simulink library "modbus_lib"  (Simulink 7.8)
settings: Solver=ode45  StartTime=0.0  StopTime=10.0  RelTol=1e-3
values from neighbouring files (symbols this model uses):
  relay_sets = xlsread('relay_settings_10272015.xlsx')    [relays_settings_init.m]
  Ts = 80e-6    (= 8e-05)    [global_parameters.m]    (also in scopeBuffer.m)
undefined symbols (not defined in the file or in its folder): angle_threshold, dF_threshold, DiscIntNeverNeededParam, dV_threshold, IOC, TOC, V, VRMSLL
libraries: simulink x24, powerlib_extras x20, powerlib x14, modbus_lib x6, simulink_extras x5, lib_Timer_Counter x4, rtio_generic_modbus x3, dspsigops x2
(part 1 of 2)
settings Model: Creator=RE25624  LastModifiedBy=re25624

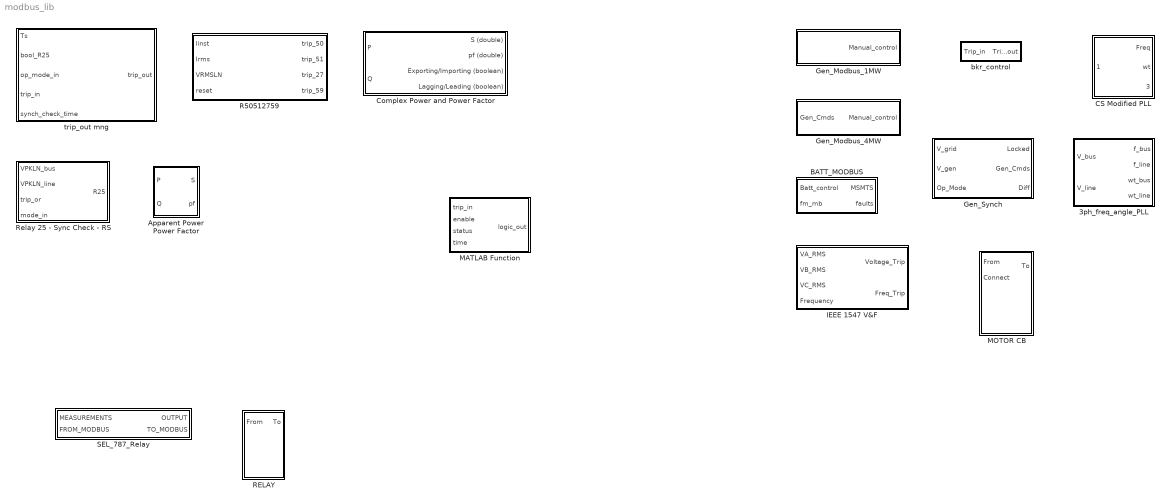
== system modbus_lib ==
  3ph_freq_angle_PLL : Subsystem
  Apparent Power Power Factor : Subsystem
  BATT_MODBUS : Subsystem
  CS Modified PLL : Subsystem  DialogController=POWERSYS.PowerSysDialog  mask(Discrete 3-phase PLL){Fmin=50, Par_Init=[0 60], ParK=[ 180 3200 1 ], Ts=Ts, AGC=off}
      mask prompts: Fmin "Minimum frequency (Hz):"; Par_Init "Initial inputs:[ Phase(degrees)   Frequency(Hz) ]"; ParK "Regulator gains [ Kp  Ki  Kd ]"; Ts "Sample time:"; AGC "Enable Automatic Gain Control"
      mask help:
      | This Phase Locked Loop (PLL) system can be used  to synchronize on a set of variable frequency, three-phase sinusoidal signals. If the Automatic Gain Control is enabled, the input (phase error) of the PLL regulator is scaled according to the input signals magnitude.
      |
      | For optimal performance, the following settings are recommended:
      |   [ Kp Ki  Kd ] = [ 180  3200  1 ]
      |   "Enable Automatic Gain Control" checked
      |
      | Input 1: Vector containing the normalized three-phase signals [Va Vb Vc]
      | Output 1:  Measured frequency (Hz) = w/(2pi)
      | Output 2:  Ramp w.t varying between  0 and 2*pi,
      |      synchronized on zero crossings of the fundamental (positive-sequence) of phase A.
      | Output 3: Vector [sin(wt) cos(wt)]
      mask init:
      | Kp=ParK(1);
      | Ki=ParK(2);
      | if length(ParK)==2
      |     Kd=0;
      | else
      |     Kd=ParK(3);
      | end    
      | Phase_Init=Par_Init(1);
      | Finit=Par_Init(2);
      | power_initmask();
      settings: OpenFcn=power_openblockproxy();
      mask Display: disp('')
  Complex Power and Power Factor : Subsystem
  Gen_Modbus_1MW : Subsystem
  Gen_Modbus_4MW : Subsystem
  Gen_Synch : Subsystem
  IEEE 1547 V&F : Subsystem  mask{V=VRMSLL, OF1=2, OF2=0.16, OV1=13, OV2=0.16, UF1=0.16, UF2=2, UV1=0.16, UV2=11, UV3=21}
      mask prompts: V "VoltageLL_RMS"; OF1 "OF1 (>60.5 Hz)"; OF2 "OF2 (>62 Hz)"; OV1 "OV1 (110% <V< 120% Vnom"; OV2 "OV2 (120% Vnom)"; UF1 "UF1 (<57 Hz)"; UF2 "UF2 (<59.5 Hz)"; UV1 "UV1 (<45% Vnom)"; UV2 "UV2 (45%<V<60% Vnom)"; UV3 "UV3 (60%<V<88% Vnom)"
      mask help:
      | This block implements interconnection system response according to IEEE Std. 1547-2014a.
      |
      | Fields to be filled are clearing times in seconds.
  MATLAB Function : MATLAB Function  TreatAsAtomicUnit=on
  MOTOR CB : Subsystem  mask(Breaker){Ts=Ts}
      mask prompts: Ts "Sampling Time [Sec]"
      mask help:
      | This block simulates the open/close behavior of a breaker. The logic (1-closed; 0-open) of operation is provided via external relay-blocks.
      | The breaker model also facilitates the system measurements for all logic functions to operate.
      | The connectivity convention adopted for this block is as follows: ABC indicates the “entry-point” or line, and the abc indicates the “exit-point” or bus.
  R50512759 : Subsystem  mask(Relays 50-51-27-59){VRMSLL=VRMSLL, IOC=IOC, TOC=TOC, Ts=Ts}
      mask prompts: VRMSLL "Nominal Voltage [VRMSLL]"; IOC "IOC Setting [A]"; TOC "TOC Setting [A]"; Ts "Sampling Time [Sec]"
      mask help:
      | This block simulates the behavior of the following relay functions:
      | 1) Instantaneous overcurrent (50)
      | 2) AC inverse time overcurrent (51)
      | 3) Undervoltage (27)
      | 4) Overvoltage (59)
      | It is not suitable for instantaneous earth current relaying.
      | The model neglects the influence CTs since only the logics of the relay are required or the current effort.
  RELAY : Subsystem  mask(Breaker){Ts=Ts}
      mask prompts: Ts "Sampling Time [Sec]"
      mask help:
      | This block simulates the open/close behavior of a breaker. The logic (1-closed; 0-open) of operation is provided via external relay-blocks.
      | The breaker model also facilitates the system measurements for all logic functions to operate.
      | The connectivity convention adopted for this block is as follows: ABC indicates the “entry-point” or line, and the abc indicates the “exit-point” or bus.
  Relay 25 - Sync Check - RS : Subsystem  mask{VRMSLL=VRMSLL, Ts=Ts, dV_threshold=dV_threshold, angle_threshold=angle_threshold, dF_threshold=dF_threshold}
      mask prompts: VRMSLL "Nominal Voltage [VRMSLL]"; Ts "Sampling Time [Sec]"; dV_threshold "Percent Voltage Threshold [%]"; angle_threshold "Angle Threshold [degress]"; dF_threshold "Frequency Threshold [Hz]"
  SEL_787_Relay : Subsystem  mask(Relay Model){bkrCtrl_enable=0, bkrCtrl_status=1, settings=[relay_sets(1, :)], Ts=Ts}
      mask prompts: bkrCtrl_enable "Enable - manual breaker control"; bkrCtrl_status "Status - manual breaker control"; settings "Relay Settings [Vnom(VRMSLL) IOC(A) TOC(A) dV(%)  dA(degrees)  dF(Hz)]"; Ts "Sampling Time [Sec]"
      mask help:
      | * The simulated relay functions are the following: synchronizing or synchronism-check (25), phase instantaneous overcurrent (50P), AC inverse time overcurrent (51P), undervoltage relay (27), and overvoltage relay (59).
      | * Modbus communication arranged to approximate SEL-787
      | * Locked-out only enabled for functions (50), (51)
      | * Over/undervoltage settings are set to +-15% of nominal voltage
      | * Manual breaker status: [1-closed, 0-open]
      mask init:
      | VRMSLL = settings(1);
      | IOC = settings(2);
      | TOC = settings(3);
      | dV_threshold = settings(4)/100;
      | angle_threshold = settings(5);
      | dF_threshold = settings(6);
  bkr_control : Subsystem  mask(Breaker control){enable=0, status=1}
      mask prompts: status "Breaker status: [1-closed, 0-open]"
      mask help: Allows the user to select which trip signal will be received at the breaker.
  trip_out mng : MATLAB Function  TreatAsAtomicUnit=on

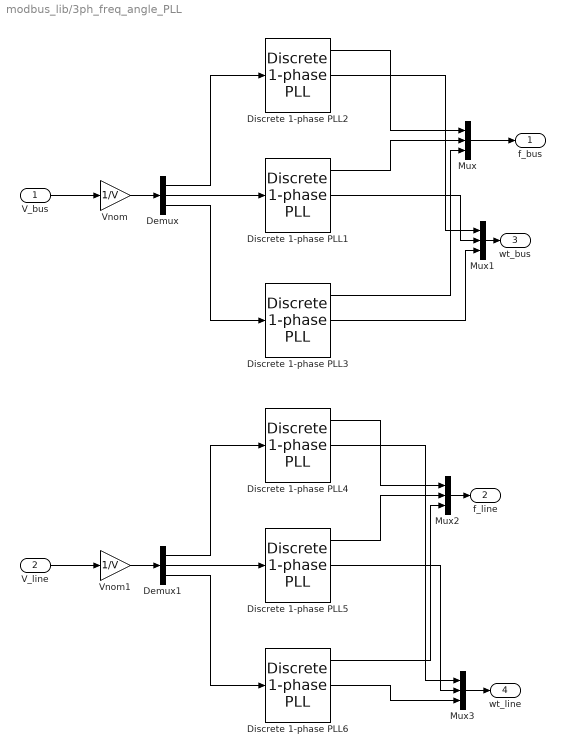
== system modbus_lib/3ph_freq_angle_PLL ==
  V_bus : Inport
  V_line : Inport  Port=2
  Demux : Demux  Outputs=3
  Demux1 : Demux  Outputs=3
  Discrete 1-phase PLL{1..6} (6 alike) : powerlib_extras/Discrete  Control Blocks/Discrete 1-phase PLL  Fmin=45  Par_Init=[0 60]  ParK=[ 180 3200 1]  Ts=50e-6  AGC=on
  Mux{,1..3} (4 alike) : Mux  Inputs=3
  Vnom : Gain  Gain=1/V
  Vnom1 : Gain  Gain=1/V
  f_bus : Outport
  f_line : Outport  Port=2
  wt_bus : Outport  Port=3
  wt_line : Outport  Port=4
  wires:
  V_bus/1 -> Vnom/1
  Mux3/1 -> wt_line/1
  Mux2/1 -> f_line/1
  Discrete 1-phase PLL6/2 -> Mux3/3
  Discrete 1-phase PLL5/2 -> Mux3/2
  Discrete 1-phase PLL4/2 -> Mux3/1
  Discrete 1-phase PLL5/1 -> Mux2/2
  Discrete 1-phase PLL6/1 -> Mux2/3
  Discrete 1-phase PLL4/1 -> Mux2/1
  Mux1/1 -> wt_bus/1
  Discrete 1-phase PLL3/2 -> Mux1/3
  Discrete 1-phase PLL1/2 -> Mux1/2
  Discrete 1-phase PLL2/2 -> Mux1/1
  Mux/1 -> f_bus/1
  Discrete 1-phase PLL3/1 -> Mux/3
  Discrete 1-phase PLL1/1 -> Mux/2
  Discrete 1-phase PLL2/1 -> Mux/1
  Demux/3 -> Discrete 1-phase PLL3/1
  Demux/2 -> Discrete 1-phase PLL1/1
  Demux/1 -> Discrete 1-phase PLL2/1
  Demux1/3 -> Discrete 1-phase PLL6/1
  Demux1/2 -> Discrete 1-phase PLL5/1
  Demux1/1 -> Discrete 1-phase PLL4/1
  Vnom1/1 -> Demux1/1
  Vnom/1 -> Demux/1
  V_line/1 -> Vnom1/1

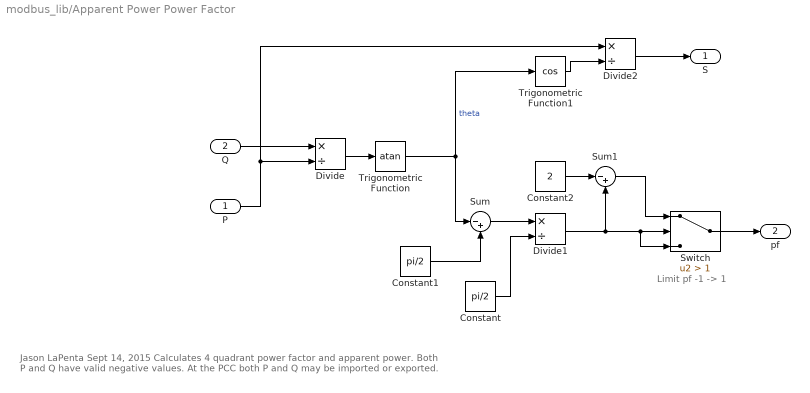
== system modbus_lib/Apparent Power Power Factor ==
  note: Limit pf -1 -> 1
  note: Jason LaPenta
      | Sept 14, 2015
      |
      | Calculates 4 quadrant power factor and apparent power.
      | Both P and Q have valid negative values. At the PCC
      | both P and Q may be imported or exported.
  P : Inport
  Q : Inport  Port=2
  Constant : Constant  Value=pi/2
  Constant1 : Constant  Value=pi/2
  Constant2 : Constant  Value=2
  Divide : Product  Inputs=*/
  Divide1 : Product  Inputs=*/
  Divide2 : Product  Inputs=*/
  Sum : Sum  Inputs=|-+
  Sum1 : Sum  Inputs=|-+
  Switch : Switch  Criteria=u2 > Threshold  Threshold=1
  Trigonometric Function : Trigonometry  Operator=atan
  Trigonometric Function1 : Trigonometry  Operator=cos
  S : Outport
  pf : Outport  Port=2
  wires:
  Switch/1 -> pf/1
  Constant2/1 -> Sum1/1
  Sum1/1 -> Switch/1
  Divide1/1 -> Switch/3, Switch/2, Sum1/2
  Sum/1 -> Divide1/1
  Constant1/1 -> Sum/2
  Divide2/1 -> S/1
  Trigonometric Function1/1 -> Divide2/2
  Constant/1 -> Divide1/2
  Trigonometric Function/1 -> Sum/1, Trigonometric Function1/1  "theta"
  Divide/1 -> Trigonometric Function/1
  P/1 -> Divide2/1, Divide/2
  Q/1 -> Divide/1

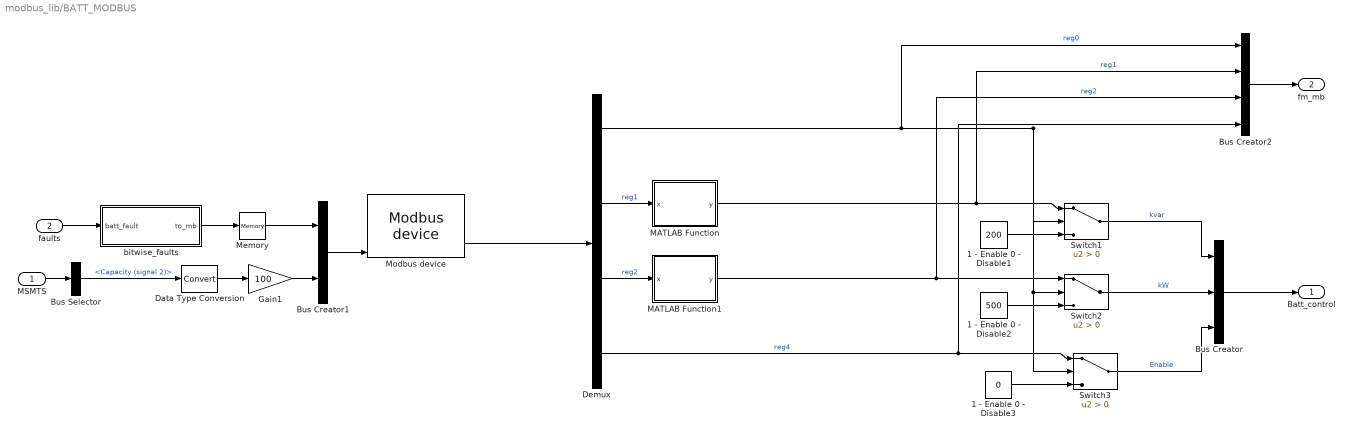
== system modbus_lib/BATT_MODBUS ==
  MSMTS : Inport
  faults : Inport  Port=2
  1 - Enable 0 - Disable1 : Constant  Value=200
  1 - Enable 0 - Disable2 : Constant  Value=500
  1 - Enable 0 - Disable3 : Constant  Value=0
  Bus Creator : BusCreator  Inputs=3
  Bus Creator1 : BusCreator  Inputs=2
  Bus Creator2 : BusCreator
  Bus Selector : BusSelector  OutputSignals=Capacity (signal 2)
  Data Type Conversion : DataTypeConversion
  Demux : Demux
  Gain1 : Gain  Gain=100
  MATLAB Function : MATLAB Function  TreatAsAtomicUnit=on
  MATLAB Function1 : MATLAB Function  TreatAsAtomicUnit=on
  Memory : Memory
  Modbus device : rtio_generic_modbus/Modbus device  conf_name=batt_slave_cfg.opal  conf_name_mask=batt_slave_cfg.xls  sample_time=Ts
  Switch1 : Switch  Criteria=u2 > Threshold
  Switch2 : Switch  Criteria=u2 > Threshold
  Switch3 : Switch  Criteria=u2 > Threshold
  bitwise_faults : Subsystem
  Batt_control : Outport
  fm_mb : Outport  Port=2
  wires:
  MATLAB Function/1(y) -> Bus Creator2/2, Switch1/1  "reg1"
  MATLAB Function1/1(y) -> Bus Creator2/3, Switch2/1  "reg2"
  Memory/1 -> Bus Creator1/1
  faults/1 -> bitwise_faults/1(batt_fault)
  bitwise_faults/1(to_mb) -> Memory/1
  Bus Creator2/1 -> fm_mb/1
  Gain1/1 -> Bus Creator1/2
  Bus Creator1/1 -> Modbus device/4
  Data Type Conversion/1 -> Gain1/1
  Bus Selector/1 -> Data Type Conversion/1  "<Capacity (signal 2)>"
  MSMTS/1 -> Bus Selector/1
  Bus Creator/1 -> Batt_control/1
  Switch3/1 -> Bus Creator/3  "Enable"
  Switch2/1 -> Bus Creator/2  "kW"
  Switch1/1 -> Bus Creator/1  "kvar"
  Demux/1 -> Bus Creator2/1, Switch3/2, Switch2/2, Switch1/2  "reg0"
  Demux/4 -> Bus Creator2/4, Switch3/1  "reg4"
  Demux/3 -> MATLAB Function1/1(x)  "reg2"
  Demux/2 -> MATLAB Function/1(x)  "reg1"
  1 - Enable 0 - Disable3/1 -> Switch3/3
  1 - Enable 0 - Disable2/1 -> Switch2/3
  1 - Enable 0 - Disable1/1 -> Switch1/3
  Modbus device/2 -> Demux/1

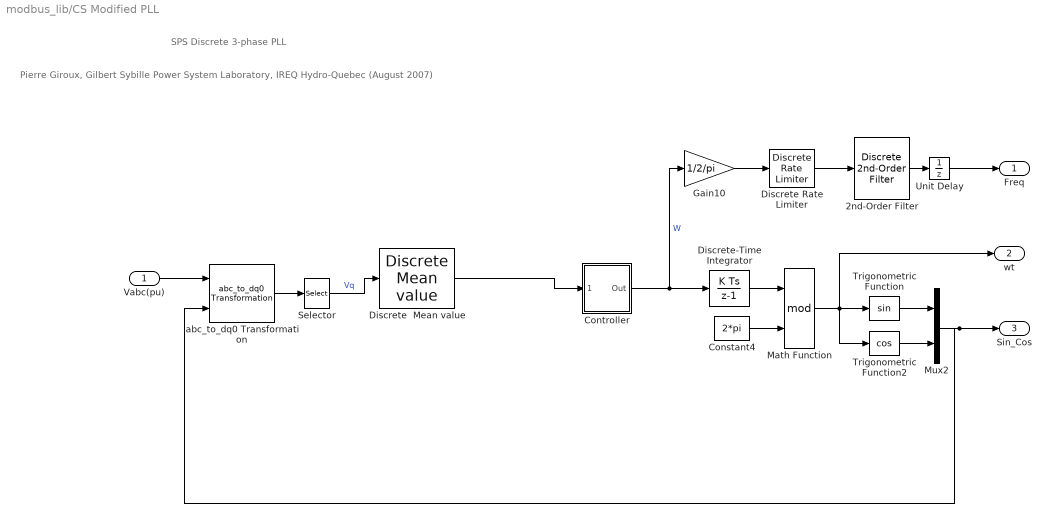
== system modbus_lib/CS Modified PLL ==
  note: Pierre Giroux, Gilbert Sybille
      | Power System Laboratory, IREQ
      | Hydro-Quebec
      | (August 2007)
  note: SPS Discrete 3-phase PLL
  Vabc(pu) : Inport  PortDimensions=3
  2nd-Order Filter : powerlib_extras/Discrete  Control Blocks/Discrete  2nd-Order Filter  FilterType=Lowpass  Fo=25  Zeta=0.707  Ts=Ts  Initialize=on  Vac_Init=[0 0 Finit]  Vdc_Init=Finit  PlotResponse=off  param1=[1 500 0.1]
  Constant4 : Constant  Value=2*pi
  Controller : Subsystem  mask(Discrete PID Controller){Kp=Kp, Ki=Ki, Kd=Kd, Par_Limits=[10000 0], Init=2*pi*Finit, Ts=Ts}
      mask prompts: Kp "Proportional gain (Kp):"; Ki "Integral gain (Ki):"; Kd "Derivative gain (Kd):"; Par_Limits "Output limits: [ Upper   Lower ]"; Init "Output initial value:"; Ts "Sample time:"
      mask help: This block implements a discrete PID controller.
      mask init:
      | UpperLimit=Par_Limits(1);
      | LowerLimit=Par_Limits(2);
      | power_initmask();
      settings: OpenFcn=power_openblockproxy();
      mask Display: disp('PID');
  Discrete Rate Limiter : powerlib_extras/Discrete  Control Blocks/Discrete Rate Limiter  R=12  F=-12  Vinit=Finit  Ts=Ts
  Discrete  Mean value : powerlib_extras/Discrete Measurements/Discrete  Mean value  Freq=60  Vinit=0  Ts=Ts
  Discrete-Time Integrator : DiscreteIntegrator  InitialCondition=Phase_Init*pi/180  SampleTime=Ts  ICPrevOutput=DiscIntNeverNeededParam  ICPrevScaledInput=DiscIntNeverNeededParam
  Gain10 : Gain  Gain=1/2/pi  SaturateOnIntegerOverflow=on  OutDataTypeStr=Inherit: Same as input  ParamDataTypeStr=Inherit: Same as input
  Math Function : Math  Operator=mod  SaturateOnIntegerOverflow=on
  Mux2 : Mux  Inputs=2
  Selector : Selector  InputPortWidth=3  IndexOptions=Index vector (dialog)  Indices=2  OutputSizes=1
  Trigonometric Function : Trigonometry
  Trigonometric Function2 : Trigonometry  Operator=cos
  Unit Delay : UnitDelay  X0=Finit  SampleTime=Ts
  abc_to_dq0 Transformation : powerlib_extras/Measurements/abc_to_dq0 Transformation
  Freq : Outport
  wt : Outport  Port=2
  Sin_Cos : Outport  Port=3
  wires:
  Selector/1 -> Discrete  Mean value/1  "Vq"
  2nd-Order Filter/1 -> Unit Delay/1
  Unit Delay/1 -> Freq/1
  Discrete Rate Limiter/1 -> 2nd-Order Filter/1
  Gain10/1 -> Discrete Rate Limiter/1
  Mux2/1 -> Sin_Cos/1, abc_to_dq0 Transformation/2
  Trigonometric Function2/1 -> Mux2/2
  Trigonometric Function/1 -> Mux2/1
  Math Function/1 -> Trigonometric Function/1, wt/1, Trigonometric Function2/1
  Discrete-Time Integrator/1 -> Math Function/1
  Constant4/1 -> Math Function/2
  abc_to_dq0 Transformation/1 -> Selector/1
  Vabc(pu)/1 -> abc_to_dq0 Transformation/1
  Controller/1(Out) -> Discrete-Time Integrator/1, Gain10/1  "W"
  Discrete  Mean value/1 -> Controller/1(Error)

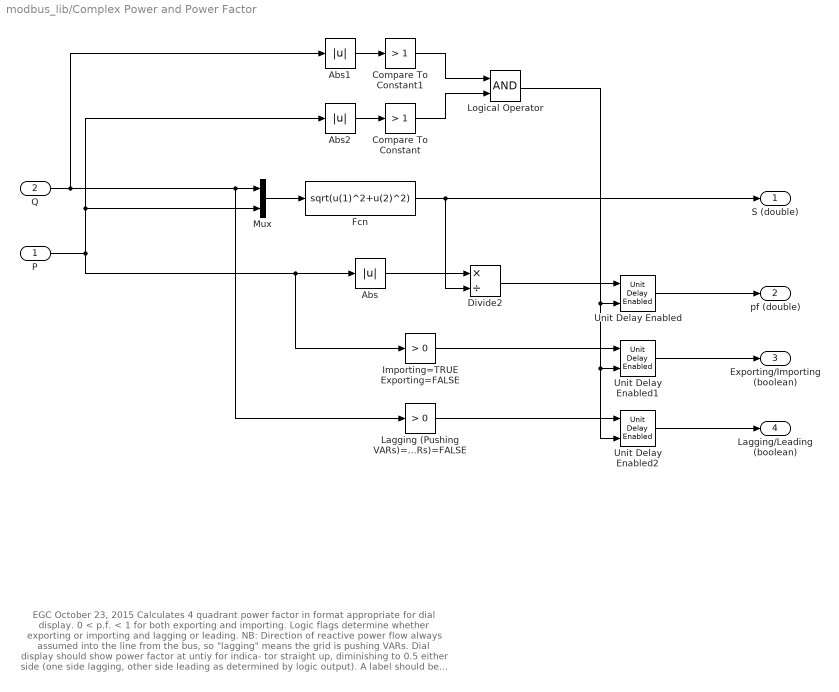
== system modbus_lib/Complex Power and Power Factor ==
  note: EGC
      | October 23, 2015
      |
      | Calculates 4 quadrant power factor in format appropriate
      | for dial display.  0 < p.f. < 1 for both exporting and
      | importing.  Logic flags determine whether exporting or
      | importing and lagging or leading.  NB:  Direction of
      | reactive power flow always assumed into the line from the
      | bus, so "lagging" means the grid is pushing VARs.
      |
      | Dial display should show power factor at untiy for indica-
      | tor straight up, diminishing to 0.5 either side (one side
      | lagging, other side leading as determined by logic output).
      | A label should be used to display EXPORTING or IMPORTING
      | based on logic output.
  P : Inport
  Q : Inport  Port=2
  Abs : Abs
  Abs1 : Abs
  Abs2 : Abs
  Compare To Constant : simulink/Logic and Bit Operations/Compare To Constant  relop=>  const=1  OutDataTypeStr=uint8
  Compare To Constant1 : simulink/Logic and Bit Operations/Compare To Constant  relop=>  const=1  OutDataTypeStr=uint8
  Divide2 : Product  Inputs=*/
  Fcn : Fcn  Expr=sqrt(u(1)^2+u(2)^2)
  Importing=TRUE Exporting=FALSE : simulink/Logic and Bit Operations/Compare To Constant  relop=>  const=0  OutDataTypeStr=boolean
  Lagging (Pushing VARs)=TRUE Leading (Pulling VARs)=FALSE : simulink/Logic and Bit Operations/Compare To Constant  relop=>  const=0  OutDataTypeStr=boolean
  Logical Operator : Logic  AllPortsSameDT=off  OutDataTypeStr=boolean
  Mux : Mux  Inputs=2
  Unit Delay Enabled : simulink/Additional Math & Discrete/Additional Discrete/Unit Delay Enabled  vinit=1  tsamp=-1
  Unit Delay Enabled1 : simulink/Additional Math & Discrete/Additional Discrete/Unit Delay Enabled  vinit=1  tsamp=-1
  Unit Delay Enabled2 : simulink/Additional Math & Discrete/Additional Discrete/Unit Delay Enabled  vinit=1  tsamp=-1
  S (double) : Outport
  pf (double) : Outport  Port=2
  Exporting/Importing (boolean) : Outport  Port=3
  Lagging/Leading (boolean) : Outport  Port=4
  wires:
  Fcn/1 -> Divide2/2, S (double)/1
  P/1 -> Abs/1, Importing=TRUE Exporting=FALSE/1, Mux/2, Abs2/1
  Q/1 -> Mux/1, Lagging (Pushing VARs)=TRUE Leading (Pulling VARs)=FALSE/1, Abs1/1
  Mux/1 -> Fcn/1
  Abs/1 -> Divide2/1
  Divide2/1 -> Unit Delay Enabled/1
  Unit Delay Enabled/1 -> pf (double)/1
  Importing=TRUE Exporting=FALSE/1 -> Unit Delay Enabled1/1
  Unit Delay Enabled1/1 -> Exporting/Importing (boolean)/1
  Lagging (Pushing VARs)=TRUE Leading (Pulling VARs)=FALSE/1 -> Unit Delay Enabled2/1
  Unit Delay Enabled2/1 -> Lagging/Leading (boolean)/1
  Abs2/1 -> Compare To Constant/1
  Abs1/1 -> Compare To Constant1/1
  Compare To Constant1/1 -> Logical Operator/1
  Compare To Constant/1 -> Logical Operator/2
  Logical Operator/1 -> Unit Delay Enabled/2, Unit Delay Enabled1/2, Unit Delay Enabled2/2

== system modbus_lib/Gen_Modbus_1MW ==
  note: This function is an attempt to substitute the switches
  Bus Creator : BusCreator  Inputs=6
  Demux : Demux  Outputs=7
  Gain : Gain  Gain=1/100
  MATLAB Function : MATLAB Function  TreatAsAtomicUnit=on
  Modbus device : rtio_generic_modbus/Modbus device  conf_name=none  conf_name_mask=gen_slave_cfg2.xls  sample_time=Ts
  Manual_control : Outport
  wires:
  Gain/1 -> Demux/1
  Modbus device/2 -> Gain/1
  Demux/1 -> MATLAB Function/1(Select_mb)
  Demux/2 -> MATLAB Function/2(P_mb)
  Demux/3 -> MATLAB Function/3(Q_mb)
  Demux/4 -> MATLAB Function/4(V_mb)
  Demux/5 -> MATLAB Function/5(F_mb)
  Demux/6 -> MATLAB Function/6(Mode_mb)
  Demux/7 -> MATLAB Function/7(Enable_mb)
  Bus Creator/1 -> Manual_control/1
  MATLAB Function/1(P) -> Bus Creator/1  "P"
  MATLAB Function/2(Q) -> Bus Creator/2  "Q"
  MATLAB Function/3(V) -> Bus Creator/3  "V"
  MATLAB Function/4(F) -> Bus Creator/4  "F"
  MATLAB Function/5(Mode) -> Bus Creator/5  "Mode"
  MATLAB Function/6(Enable) -> Bus Creator/6  "Enable"

== system modbus_lib/Gen_Modbus_4MW ==
  note: This function is an attempt to substitute the switches
  Gen_Cmds : Inport
  Bus Creator : BusCreator  Inputs=6
  Demux : Demux  Outputs=7
  Gain : Gain  Gain=1/100
  MATLAB Function : MATLAB Function  TreatAsAtomicUnit=on
  Modbus device : rtio_generic_modbus/Modbus device  conf_name=gen_slave_cfg.opal  conf_name_mask=gen_slave_cfg.xls  sample_time=Ts
  Manual_control : Outport
  wires:
  Gain/1 -> Demux/1
  Demux/1 -> MATLAB Function/1(Select_mb)
  Demux/2 -> MATLAB Function/2(P_mb)
  Demux/3 -> MATLAB Function/3(Q_mb)
  Demux/4 -> MATLAB Function/4(V_mb)
  Demux/5 -> MATLAB Function/5(F_mb)
  Demux/6 -> MATLAB Function/6(Mode_mb)
  Demux/7 -> MATLAB Function/7(Enable_mb)
  Bus Creator/1 -> Manual_control/1
  MATLAB Function/1(P) -> Bus Creator/1  "P"
  MATLAB Function/2(Q) -> Bus Creator/2  "Q"
  MATLAB Function/3(V) -> Bus Creator/3  "V"
  MATLAB Function/4(F) -> Bus Creator/4  "F"
  MATLAB Function/5(Mode) -> Bus Creator/5  "Mode"
  MATLAB Function/6(Enable) -> Bus Creator/6  "Enable"
  Modbus device/2 -> Gain/1
  Gen_Cmds/1 -> MATLAB Function/8(gen_cmds)

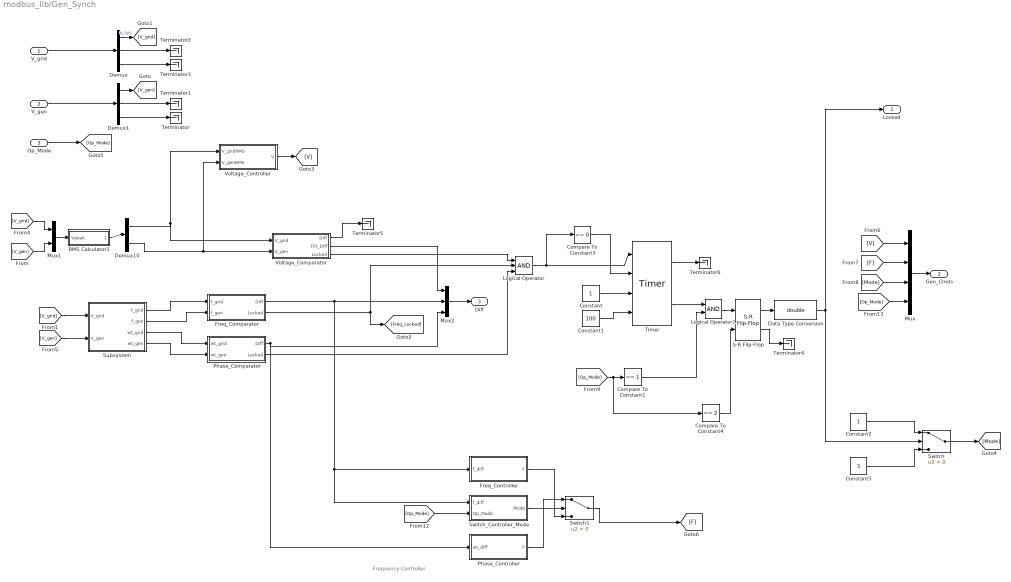
== system modbus_lib/Gen_Synch ==
  note: Frequency Controller
  V_grid : Inport
  V_gen : Inport  Port=2
  Op_Mode : Inport  Port=3
  Compare To Constant1 : simulink/Logic and Bit Operations/Compare To Constant  relop===  const=1  OutDataTypeStr=boolean
  Compare To Constant3 : simulink/Logic and Bit Operations/Compare To Constant  relop===  const=0  OutDataTypeStr=uint8
  Compare To Constant4 : simulink/Logic and Bit Operations/Compare To Constant  relop===  const=2  OutDataTypeStr=boolean
  Constant : Constant
  Constant1 : Constant  Value=100
  Constant2 : Constant
  Constant3 : Constant  Value=3
  Data Type Conversion : DataTypeConversion  OutDataTypeStr=double
  Demux : Demux  Outputs=3
  Demux1 : Demux  Outputs=3
  Demux10 : Demux  Outputs=2
  Freq_Comparator : Subsystem
  Freq_Controller : Subsystem
  Logical Operator : Logic  Inputs=3  AllPortsSameDT=off  OutDataTypeStr=boolean
  Logical Operator1 : Logic  AllPortsSameDT=off  OutDataTypeStr=boolean
  Mux : Mux
  Mux1 : Mux  Inputs=2
  Mux2 : Mux  Inputs=3
  Phase_Comparator : Subsystem
  Phase_Controller : Subsystem
  RMS Calculator3 : Subsystem
  S-R Flip-Flop : simulink_extras/Flip Flops/S-R Flip-Flop  initial_condition=0
  Subsystem : Subsystem
  Switch : Switch  Criteria=u2 > Threshold
  Switch1 : Switch  Criteria=u2 > Threshold
  Switch_Controller_Mode : Subsystem
  Terminator{,1..6} (7 alike) : Terminator
  Timer : lib_Timer_Counter/Timer
  Voltage_Comparator : Subsystem
  Voltage_Controller : Subsystem
  Locked : Outport
  Gen_Cmds : Outport  Port=2  PortDimensions=4
  Diff : Outport  Port=3
  wires:
  Phase_Comparator/1(Diff) -> Mux2/3, Phase_Controller/1(wt_diff)
  Freq_Comparator/1(Diff) -> Mux2/2, Freq_Controller/1(f_diff), Switch_Controller_Mode/1(f_diff)
  Voltage_Comparator/2(Filt_Diff) -> Mux2/1
  [V_gen] -> Subsystem/2(V_gen)
  [V_grid] -> Subsystem/1(V_grid)
  Demux/1 -> [V_grid]  "a_sys"
  Demux1/1 -> [V_gen]
  Data Type Conversion/1 -> Switch/2, Locked/1
  S-R Flip-Flop/1 -> Data Type Conversion/1
  Logical Operator/1 -> Compare To Constant3/1, Timer/1
  Compare To Constant3/1 -> Timer/2
  Constant1/1 -> Timer/4
  Constant/1 -> Timer/3
  Phase_Comparator/2(Locked) -> Logical Operator/3
  Freq_Comparator/2(Locked) -> Logical Operator/2, [Freq_Locked]
  Voltage_Comparator/3(Locked) -> Logical Operator/1
  Subsystem/4(wt_gen) -> Phase_Comparator/2(wt_gen)
  Subsystem/3(wt_grid) -> Phase_Comparator/1(wt_grid)
  Subsystem/2(f_gen) -> Freq_Comparator/2(f_gen)
  Subsystem/1(f_grid) -> Freq_Comparator/1(f_grid)
  V_gen/1 -> Demux1/1
  V_grid/1 -> Demux/1
  Constant2/1 -> Switch/1
  Constant3/1 -> Switch/3
  Switch/1 -> [Mode]
  Mux/1 -> Gen_Cmds/1
  [V] -> Mux/1
  [Mode] -> Mux/3
  [F] -> Mux/2
  Timer/2 -> Logical Operator1/1
  Compare To Constant1/1 -> Logical Operator1/2
  Mux2/1 -> Diff/1
  Switch1/1 -> [F]
  Switch_Controller_Mode/1(Mode) -> Switch1/2
  Op_Mode/1 -> [Op_Mode]
  [Op_Mode] -> Compare To Constant1/1, Compare To Constant4/1
  Logical Operator1/1 -> S-R Flip-Flop/1
  Compare To Constant4/1 -> S-R Flip-Flop/2
  [Op_Mode] -> Mux/4
  Voltage_Controller/1(V) -> [V]
  Freq_Controller/1(F) -> Switch1/3
  Phase_Controller/1(F) -> Switch1/1
  [Op_Mode] -> Switch_Controller_Mode/2(Op_Mode)
  Demux1/2 -> Terminator1/1
  Demux1/3 -> Terminator/1
  Demux/2 -> Terminator2/1
  Demux/3 -> Terminator3/1
  S-R Flip-Flop/2 -> Terminator4/1
  Voltage_Comparator/1(Diff) -> Terminator5/1
  Demux10/2 -> Voltage_Comparator/2(V_gen), Voltage_Controller/2(V_genRMS)
  Mux1/1 -> RMS Calculator3/1(Vpeak)
  RMS Calculator3/1(VRMSLL) -> Demux10/1
  [V_grid] -> Mux1/1
  [V_gen] -> Mux1/2
  Demux10/1 -> Voltage_Controller/1(V_gridRMS), Voltage_Comparator/1(V_grid)
  Timer/1 -> Terminator6/1

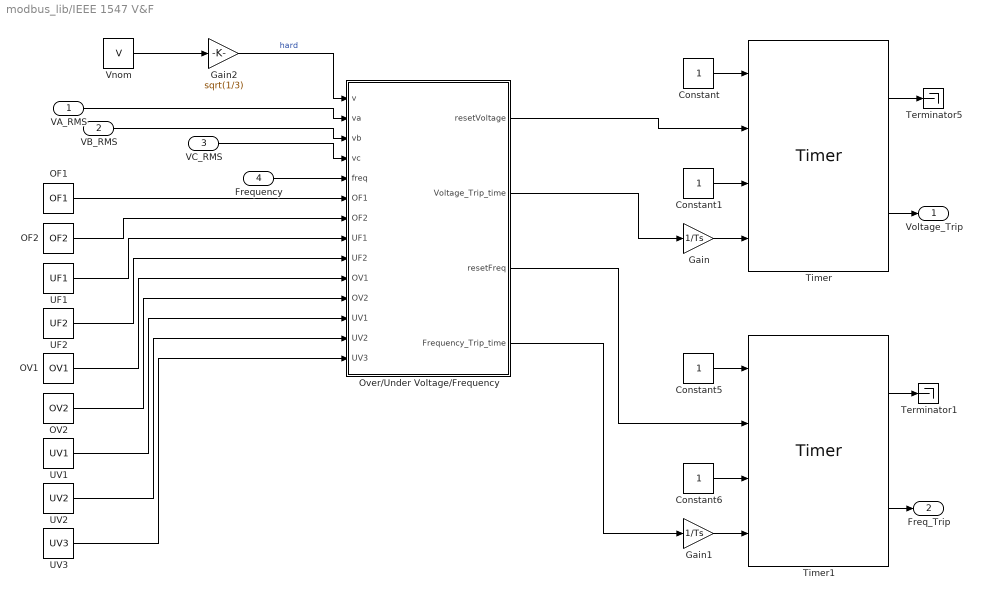
== system modbus_lib/IEEE 1547 V&F ==
  VA_RMS : Inport
  VB_RMS : Inport  Port=2
  VC_RMS : Inport  Port=3
  Frequency : Inport  Port=4
  Constant{,1,5..6} (4 alike) : Constant
  Gain : Gain  Gain=1/Ts
  Gain1 : Gain  Gain=1/Ts
  Gain2 : Gain  Gain=sqrt(1/3)
  OF1 : Constant  Value=OF1
  OF2 : Constant  Value=OF2
  OV1 : Constant  Value=OV1
  OV2 : Constant  Value=OV2
  Over/Under Voltage/Frequency : MATLAB Function  TreatAsAtomicUnit=on
  Terminator1 : Terminator
  Terminator5 : Terminator
  Timer : lib_Timer_Counter/Timer
  Timer1 : lib_Timer_Counter/Timer
  UF1 : Constant  Value=UF1
  UF2 : Constant  Value=UF2
  UV1 : Constant  Value=UV1
  UV2 : Constant  Value=UV2
  UV3 : Constant  Value=UV3
  Vnom : Constant  Value=V
  Voltage_Trip : Outport
  Freq_Trip : Outport  Port=2
  wires:
  UV3/1 -> Over/Under Voltage/Frequency/14(UV3)
  UV2/1 -> Over/Under Voltage/Frequency/13(UV2)
  UV1/1 -> Over/Under Voltage/Frequency/12(UV1)
  OV2/1 -> Over/Under Voltage/Frequency/11(OV2)
  OV1/1 -> Over/Under Voltage/Frequency/10(OV1)
  UF2/1 -> Over/Under Voltage/Frequency/9(UF2)
  UF1/1 -> Over/Under Voltage/Frequency/8(UF1)
  OF2/1 -> Over/Under Voltage/Frequency/7(OF2)
  OF1/1 -> Over/Under Voltage/Frequency/6(OF1)
  Gain/1 -> Timer/4
  Gain1/1 -> Timer1/4
  Frequency/1 -> Over/Under Voltage/Frequency/5(freq)
  VC_RMS/1 -> Over/Under Voltage/Frequency/4(vc)
  VB_RMS/1 -> Over/Under Voltage/Frequency/3(vb)
  Vnom/1 -> Gain2/1
  VA_RMS/1 -> Over/Under Voltage/Frequency/2(va)
  Timer1/2 -> Freq_Trip/1
  Constant6/1 -> Timer1/3
  Constant5/1 -> Timer1/1
  Constant1/1 -> Timer/3
  Constant/1 -> Timer/1
  Timer1/1 -> Terminator1/1
  Timer/1 -> Terminator5/1
  Timer/2 -> Voltage_Trip/1
  Over/Under Voltage/Frequency/1(resetVoltage) -> Timer/2
  Over/Under Voltage/Frequency/2(Voltage_Trip_time) -> Gain/1
  Over/Under Voltage/Frequency/4(Frequency_Trip_time) -> Gain1/1
  Over/Under Voltage/Frequency/3(resetFreq) -> Timer1/2
  Gain2/1 -> Over/Under Voltage/Frequency/1(v)  "hard"

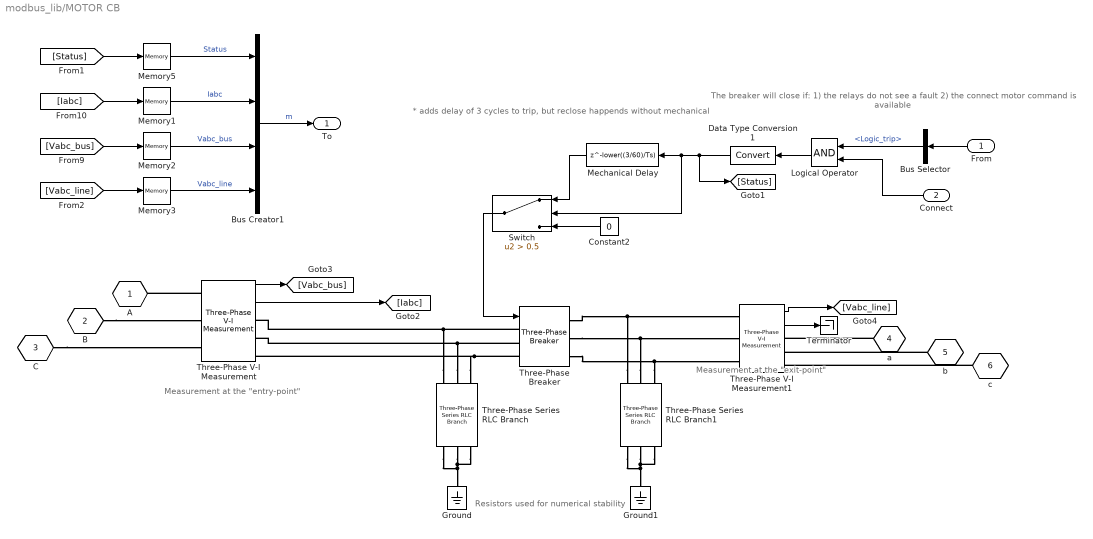
== system modbus_lib/MOTOR CB ==
  note: * adds delay of 3 cycles to trip, but reclose happends without mechanical
  note: Measurement at the "exit-point"
  note: Measurement at the "entry-point"
  note: Resistors used for numerical stability
  note: The breaker will close if:
      | 1) the relays do not see a fault
      | 2) the connect motor command is available
  From : Inport
  Connect : Inport  Port=2
  Bus Creator1 : BusCreator
  Bus Selector : BusSelector  OutputSignals=Logic_trip
  Constant2 : Constant  Value=0
  Data Type Conversion1 : DataTypeConversion
  Ground : powerlib/Elements/Ground  LConnTagsString=a
  Ground1 : powerlib/Elements/Ground  LConnTagsString=a
  Logical Operator : Logic  AllPortsSameDT=off  OutDataTypeStr=boolean
  Mechanical Delay : Delay  DelayLength=lower((3/60)/Ts)  InitialCondition=1
  Memory{1..3,5} (4 alike) : Memory
  Switch : Switch  Criteria=u2 > Threshold  Threshold=0.5
  Terminator : Terminator
  Three-Phase Series RLC Branch : powerlib/Elements/Three-Phase Series RLC Branch  LConnTagsString=A|B|C  RConnTagsString=A|B|C  BranchType=R  Resistance=15E6  Inductance=1e-3  Capacitance=1e-6  Measurements=None
  Three-Phase Series RLC Branch1 : powerlib/Elements/Three-Phase Series RLC Branch  LConnTagsString=A|B|C  RConnTagsString=A|B|C  BranchType=R  Resistance=15E6  Inductance=1e-3  Capacitance=1e-6  Measurements=None
  Three-Phase V-I Measurement : powerlib/Measurements/Three-Phase V-I Measurement  VoltageMeasurement=phase-to-ground  SetLabelV=off  LabelV=Vabc  Vpu=off  VpuLL=off  CurrentMeasurement=yes  SetLabelI=off  LabelI=Iabc  Ipu=off  Pbase=100e6  Vbase=500e3  OutputType=Complex  PhasorSimulation=off  PSBequivalent=0
  Three-Phase V-I Measurement1 : powerlib/Measurements/Three-Phase V-I Measurement  VoltageMeasurement=phase-to-ground  SetLabelV=off  LabelV=Vabc  Vpu=off  VpuLL=off  CurrentMeasurement=yes  SetLabelI=off  LabelI=Iabc  Ipu=off  Pbase=100e6  Vbase=500e3  OutputType=Complex  PhasorSimulation=off  PSBequivalent=0
  Three-Phase Breaker : powerlib/Elements/Three-Phase Breaker  InitialState=open  SwitchA=on  SwitchB=on  SwitchC=on  SwitchTimes="[1/60  5/60]"  External=on  BreakerResistance=1e-4  SnubberResistance=1E15  SnubberCapacitance=inf  Measurements=None
  A : PMIOPort  Tag=PMCPort  Port=1  Side=Left
  B : PMIOPort  Tag=PMCPort  Port=2  Side=Left
  C : PMIOPort  Tag=PMCPort  Port=3  Side=Left
  a : PMIOPort  Tag=PMCPort  Port=4  Side=Right
  b : PMIOPort  Tag=PMCPort  Port=5  Side=Right
  c : PMIOPort  Tag=PMCPort  Port=6  Side=Right
  To : Outport
  wires:
  Constant2/1 -> Switch/3
  Mechanical Delay/1 -> Switch/1
  Switch/1 -> Three-Phase Breaker/1
  Memory3/1 -> Bus Creator1/4  "Vabc_line"
  Memory2/1 -> Bus Creator1/3  "Vabc_bus"
  Memory1/1 -> Bus Creator1/2  "Iabc"
  Memory5/1 -> Bus Creator1/1  "Status"
  Three-Phase V-I Measurement1/2 -> Terminator/1
  [Vabc_line] -> Memory3/1
  Three-Phase V-I Measurement1/1 -> [Vabc_line]
  From/1 -> Bus Selector/1
  [Vabc_bus] -> Memory2/1
  [Iabc] -> Memory1/1
  [Status] -> Memory5/1
  Data Type Conversion1/1 -> Switch/2, Mechanical Delay/1, [Status]
  Three-Phase V-I Measurement/2 -> [Iabc]
  Three-Phase V-I Measurement/1 -> [Vabc_bus]
  Bus Creator1/1 -> To/1  "m"
  Logical Operator/1 -> Data Type Conversion1/1
  Bus Selector/1 -> Logical Operator/1  "<Logic_trip>"
  Connect/1 -> Logical Operator/2
  connections:
  Three-Phase Series RLC Branch1/RConn1 -- Ground1/LConn1 -- Three-Phase Series RLC Branch1/RConn3 -- Three-Phase Series RLC Branch1/RConn2
  Three-Phase Series RLC Branch/RConn1 -- Ground/LConn1 -- Three-Phase Series RLC Branch/RConn3 -- Three-Phase Series RLC Branch/RConn2
  Three-Phase Series RLC Branch/LConn1 -- Three-Phase V-I Measurement/RConn1 -- Three-Phase Breaker/LConn1
  Three-Phase Series RLC Branch/LConn2 -- Three-Phase V-I Measurement/RConn2 -- Three-Phase Breaker/LConn2
  Three-Phase Series RLC Branch/LConn3 -- Three-Phase V-I Measurement/RConn3 -- Three-Phase Breaker/LConn3
  Three-Phase Series RLC Branch1/LConn1 -- Three-Phase V-I Measurement1/LConn1 -- Three-Phase Breaker/RConn1
  Three-Phase Series RLC Branch1/LConn2 -- Three-Phase V-I Measurement1/LConn2 -- Three-Phase Breaker/RConn2
  Three-Phase Series RLC Branch1/LConn3 -- Three-Phase V-I Measurement1/LConn3 -- Three-Phase Breaker/RConn3
  Three-Phase V-I Measurement/LConn1 -- A/RConn1
  B/RConn1 -- Three-Phase V-I Measurement/LConn2
  C/RConn1 -- Three-Phase V-I Measurement/LConn3
  a/RConn1 -- Three-Phase V-I Measurement1/RConn1
  b/RConn1 -- Three-Phase V-I Measurement1/RConn2
  c/RConn1 -- Three-Phase V-I Measurement1/RConn3

== system modbus_lib/R50512759 ==
  Iinst : Inport
  Irms : Inport  Port=2
  VRMSLN : Inport  Port=3
  reset : Inport  Port=4
  Data Type Conversion3 : DataTypeConversion
  Relays : MATLAB Function  TreatAsAtomicUnit=on
  a1 : Constant  Value=VRMSLL
  a2 : Constant  Value=TOC
  a4 : Constant  Value=Ts
  a5 : Constant  Value=IOC
  trip_50 : Outport
  trip_51 : Outport  Port=2
  trip_27 : Outport  Port=3
  trip_59 : Outport  Port=4
  wires:
  reset/1 -> Data Type Conversion3/1
  a5/1 -> Relays/6(IOC)  "IOC"
  Iinst/1 -> Relays/3(Iinst)
  a2/1 -> Relays/7(TOC)  "TOC"
  Irms/1 -> Relays/4(Irms)
  VRMSLN/1 -> Relays/5(Vrms)
  a1/1 -> Relays/8(VRMSLL)  "VRMSLL"
  a4/1 -> Relays/1(Ts)
  Relays/3(trip27) -> trip_27/1  "t27"
  Relays/4(trip59) -> trip_59/1  "t59"
  Relays/1(trip50) -> trip_50/1  "t50"
  Relays/2(trip51) -> trip_51/1  "t51"
  Data Type Conversion3/1 -> Relays/2(Reset)

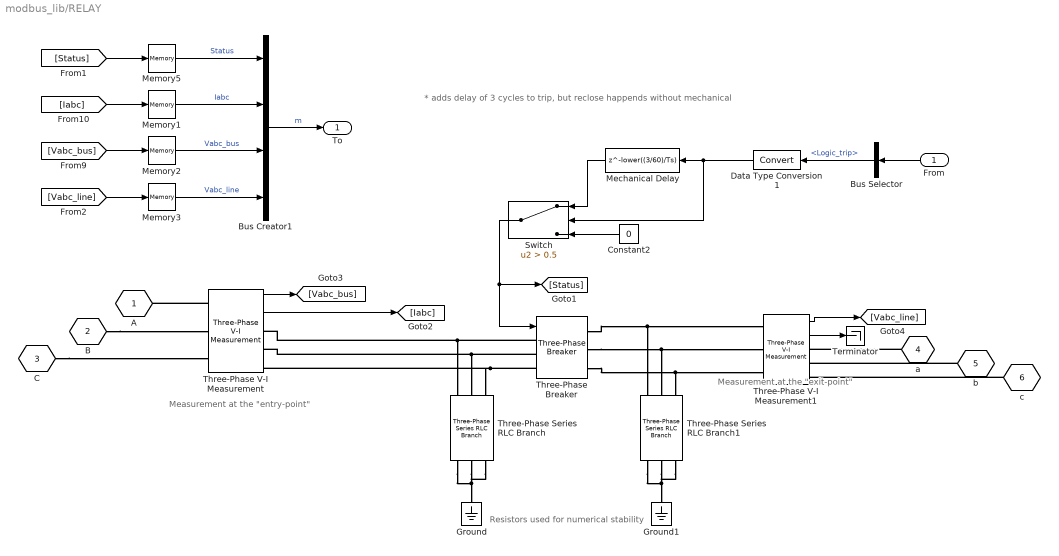
== system modbus_lib/RELAY ==
  note: Resistors used for numerical stability
  note: Measurement at the "entry-point"
  note: Measurement at the "exit-point"
  note: * adds delay of 3 cycles to trip, but reclose happends without mechanical
  From : Inport
  Bus Creator1 : BusCreator
  Bus Selector : BusSelector  OutputSignals=Logic_trip
  Constant2 : Constant  Value=0
  Data Type Conversion1 : DataTypeConversion
  Ground : powerlib/Elements/Ground  LConnTagsString=a
  Ground1 : powerlib/Elements/Ground  LConnTagsString=a
  Mechanical Delay : Delay  DelayLength=lower((3/60)/Ts)  InitialCondition=1
  Memory{1..3,5} (4 alike) : Memory
  Switch : Switch  Criteria=u2 > Threshold  Threshold=0.5
  Terminator : Terminator
  Three-Phase Series RLC Branch : powerlib/Elements/Three-Phase Series RLC Branch  LConnTagsString=A|B|C  RConnTagsString=A|B|C  BranchType=R  Resistance=15E6  Inductance=1e-3  Capacitance=1e-6  Measurements=None
  Three-Phase Series RLC Branch1 : powerlib/Elements/Three-Phase Series RLC Branch  LConnTagsString=A|B|C  RConnTagsString=A|B|C  BranchType=R  Resistance=15E6  Inductance=1e-3  Capacitance=1e-6  Measurements=None
  Three-Phase V-I Measurement : powerlib/Measurements/Three-Phase V-I Measurement  VoltageMeasurement=phase-to-ground  SetLabelV=off  LabelV=Vabc  Vpu=off  VpuLL=off  CurrentMeasurement=yes  SetLabelI=off  LabelI=Iabc  Ipu=off  Pbase=100e6  Vbase=500e3  OutputType=Complex  PhasorSimulation=off  PSBequivalent=0
  Three-Phase V-I Measurement1 : powerlib/Measurements/Three-Phase V-I Measurement  VoltageMeasurement=phase-to-ground  SetLabelV=off  LabelV=Vabc  Vpu=off  VpuLL=off  CurrentMeasurement=yes  SetLabelI=off  LabelI=Iabc  Ipu=off  Pbase=100e6  Vbase=500e3  OutputType=Complex  PhasorSimulation=off  PSBequivalent=0
  Three-Phase Breaker : powerlib/Elements/Three-Phase Breaker  InitialState=closed  SwitchA=on  SwitchB=on  SwitchC=on  SwitchTimes="[1/60  5/60]"  External=on  BreakerResistance=1e-4  SnubberResistance=1E15  SnubberCapacitance=inf  Measurements=None
  A : PMIOPort  Tag=PMCPort  Port=1  Side=Left
  B : PMIOPort  Tag=PMCPort  Port=2  Side=Left
  C : PMIOPort  Tag=PMCPort  Port=3  Side=Left
  a : PMIOPort  Tag=PMCPort  Port=4  Side=Right
  b : PMIOPort  Tag=PMCPort  Port=5  Side=Right
  c : PMIOPort  Tag=PMCPort  Port=6  Side=Right
  To : Outport
  wires:
  Bus Creator1/1 -> To/1  "m"
  Three-Phase V-I Measurement/1 -> [Vabc_bus]
  Three-Phase V-I Measurement/2 -> [Iabc]
  Data Type Conversion1/1 -> Mechanical Delay/1, Switch/2
  [Status] -> Memory5/1
  [Iabc] -> Memory1/1
  [Vabc_bus] -> Memory2/1
  From/1 -> Bus Selector/1
  Three-Phase V-I Measurement1/1 -> [Vabc_line]
  [Vabc_line] -> Memory3/1
  Three-Phase V-I Measurement1/2 -> Terminator/1
  Memory5/1 -> Bus Creator1/1  "Status"
  Memory1/1 -> Bus Creator1/2  "Iabc"
  Memory2/1 -> Bus Creator1/3  "Vabc_bus"
  Memory3/1 -> Bus Creator1/4  "Vabc_line"
  Bus Selector/1 -> Data Type Conversion1/1  "<Logic_trip>"
  Switch/1 -> Three-Phase Breaker/1, [Status]
  Mechanical Delay/1 -> Switch/1
  Constant2/1 -> Switch/3
  connections:
  c/RConn1 -- Three-Phase V-I Measurement1/RConn3
  b/RConn1 -- Three-Phase V-I Measurement1/RConn2
  a/RConn1 -- Three-Phase V-I Measurement1/RConn1
  C/RConn1 -- Three-Phase V-I Measurement/LConn3
  B/RConn1 -- Three-Phase V-I Measurement/LConn2
  Three-Phase V-I Measurement/LConn1 -- A/RConn1
  Three-Phase Breaker/RConn3 -- Three-Phase V-I Measurement1/LConn3 -- Three-Phase Series RLC Branch1/LConn3
  Three-Phase Breaker/RConn2 -- Three-Phase V-I Measurement1/LConn2 -- Three-Phase Series RLC Branch1/LConn2
  Three-Phase Breaker/RConn1 -- Three-Phase V-I Measurement1/LConn1 -- Three-Phase Series RLC Branch1/LConn1
  Three-Phase Breaker/LConn3 -- Three-Phase V-I Measurement/RConn3 -- Three-Phase Series RLC Branch/LConn3
  Three-Phase Breaker/LConn2 -- Three-Phase V-I Measurement/RConn2 -- Three-Phase Series RLC Branch/LConn2
  Three-Phase Breaker/LConn1 -- Three-Phase V-I Measurement/RConn1 -- Three-Phase Series RLC Branch/LConn1
  Three-Phase Series RLC Branch/RConn2 -- Three-Phase Series RLC Branch/RConn3 -- Ground/LConn1 -- Three-Phase Series RLC Branch/RConn1
  Three-Phase Series RLC Branch1/RConn2 -- Three-Phase Series RLC Branch1/RConn3 -- Ground1/LConn1 -- Three-Phase Series RLC Branch1/RConn1

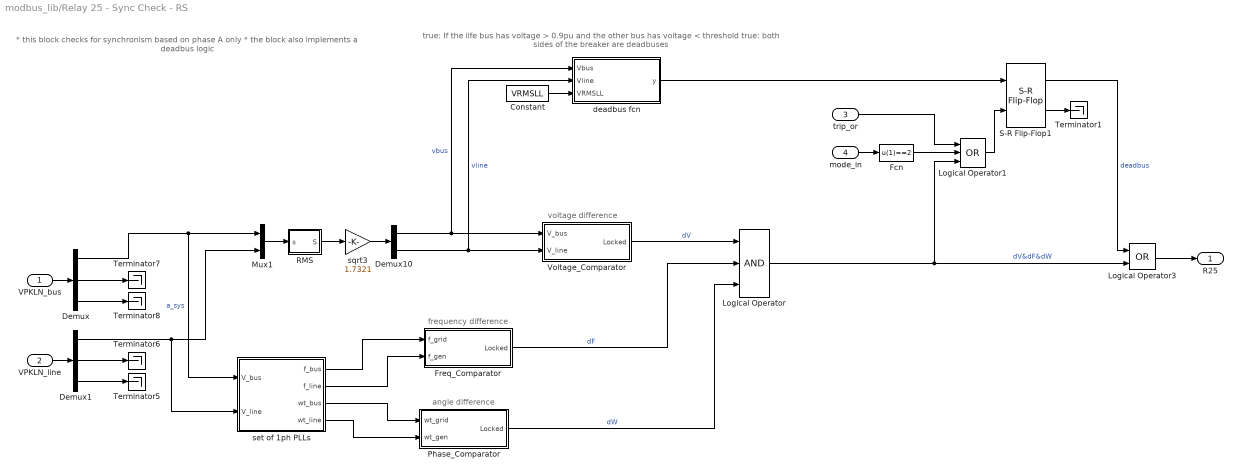
== system modbus_lib/Relay 25 - Sync Check - RS ==
  note: true: If the life bus has voltage > 0.9pu and the other bus has voltage < threshold
      | true: both sides of the breaker are deadbuses
  note: voltage difference
  note: frequency difference
  note: angle difference
  note: * this block checks for synchronism based on phase A only
      | * the block also implements a deadbus logic
  VPKLN_bus : Inport
  VPKLN_line : Inport  Port=2
  trip_or : Inport  Port=3
  mode_in : Inport  Port=4
  Constant : Constant  Value=VRMSLL
  Demux : Demux  Outputs=3
  Demux1 : Demux  Outputs=3
  Demux10 : Demux  Outputs=2
  Fcn : Fcn  Expr=u(1)==2
  Freq_Comparator : Subsystem
  Logical Operator : Logic  Inputs=3  AllPortsSameDT=off  OutDataTypeStr=boolean
  Logical Operator1 : Logic  Operator=OR  Inputs=3  AllPortsSameDT=off  OutDataTypeStr=boolean
  Logical Operator3 : Logic  Operator=OR  AllPortsSameDT=off  OutDataTypeStr=boolean
  Mux1 : Mux  Inputs=2
  Phase_Comparator : Subsystem
  RMS : Subsystem
  S-R Flip-Flop1 : simulink_extras/Flip Flops/S-R Flip-Flop  initial_condition=0
  Terminator{1,5..8} (5 alike) : Terminator
  Voltage_Comparator : Subsystem
  deadbus fcn : MATLAB Function  TreatAsAtomicUnit=on
  set of 1ph PLLs : Subsystem
  sqrt3 : Gain  Gain=1.7321
  R25 : Outport
  wires:
  Logical Operator/1 -> Logical Operator3/2, Logical Operator1/3  "dV&dF&dW"
  VPKLN_line/1 -> Demux1/1
  VPKLN_bus/1 -> Demux/1
  Demux/3 -> Terminator8/1
  Demux/2 -> Terminator7/1
  Demux1/3 -> Terminator5/1
  Demux1/2 -> Terminator6/1
  Demux1/1 -> set of 1ph PLLs/2(V_line), Mux1/2
  Demux/1 -> set of 1ph PLLs/1(V_bus), Mux1/1  "a_sys"
  Demux10/1 -> Voltage_Comparator/1(V_bus), deadbus fcn/1(Vbus)  "vbus"
  set of 1ph PLLs/1(f_bus) -> Freq_Comparator/1(f_grid)
  set of 1ph PLLs/2(f_line) -> Freq_Comparator/2(f_gen)
  set of 1ph PLLs/3(wt_bus) -> Phase_Comparator/1(wt_grid)
  set of 1ph PLLs/4(wt_line) -> Phase_Comparator/2(wt_gen)
  Demux10/2 -> Voltage_Comparator/2(V_line), deadbus fcn/2(Vline)  "vline"
  Voltage_Comparator/1(Locked) -> Logical Operator/1  "dV"
  Freq_Comparator/1(Locked) -> Logical Operator/2  "dF"
  Phase_Comparator/1(Locked) -> Logical Operator/3  "dW"
  RMS/1(S) -> sqrt3/1
  Mux1/1 -> RMS/1(s)
  sqrt3/1 -> Demux10/1
  Constant/1 -> deadbus fcn/3(VRMSLL)
  S-R Flip-Flop1/2 -> Terminator1/1
  Logical Operator3/1 -> R25/1
  S-R Flip-Flop1/1 -> Logical Operator3/1  "deadbus"
  deadbus fcn/1(y) -> S-R Flip-Flop1/1
  Logical Operator1/1 -> S-R Flip-Flop1/2
  trip_or/1 -> Logical Operator1/1
  mode_in/1 -> Fcn/1
  Fcn/1 -> Logical Operator1/2

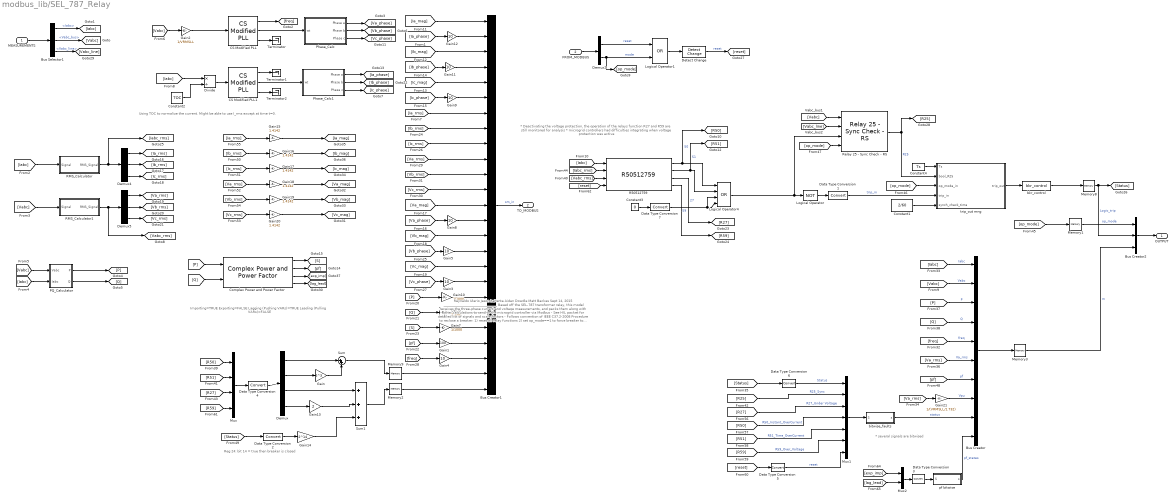
== system modbus_lib/SEL_787_Relay ==
  note: Reynaldo Ulerio
      | Jason LaPenta
      | Aidan Dowdle
      | Matt Backes
      | Sept 14, 2015
      | ________________________________
      |
      | Based off the SEL-787 transformer relay, this model receives
      | the three-phase current and voltage measurements, and packs
      | them along with other calculations to send to the microgrid
      | controller via Modbus
      |
      | - See HIL packet for detailed list of signals and scale factors
      | - Follows convention of IEEE C37.2-2008
      |
      | Procedure to reclose a breaker:
      | 1) reset all relay functions
      | 2) set op_mode==1 to force breaker to close
      |    --> The relay function 25 will automatically activate
      | 3) change op_mode==0 for logic based operation
  note: Reg 24: bit 14 = true then breaker is closed
  note: Using TOC to normalize the current. Might be able to use I_rms except at time t=0.
  note: * several signals are bitwised
  note: Importing=TRUE
      | Exporting=FALSE
      |
      | Lagging (Pushing VARs)=TRUE
      | Leading (Pulling VARs)=FALSE
  note: * Deactivating the voltage protection, the operation of the relays function
      |  R27 and R59 are still monitored for analysis
      |
      | * microgrid controllers had difficulties integrating when voltage protection was active
  MEASUREMENTS : Inport
  FROM_MODBUS : Inport  Port=2
  Bus Creator : BusCreator  Inputs=10
  Bus Creator1 : BusCreator  Inputs=25
  Bus Creator2 : BusCreator  Inputs=3
  Bus Selector1 : BusSelector  OutputSignals=Iabc,Vabc_bus,Vabc_line
  CS Modified PLL : modbus_lib/CS Modified PLL  Fmin=50  Par_Init=[0 60]  ParK=[ 180 3200 1 ]  Ts=Ts  AGC=off
  CS Modified PLL1 : modbus_lib/CS Modified PLL  Fmin=50  Par_Init=[0 60]  ParK=[ 180 3200 1 ]  Ts=Ts  AGC=off
  Complex Power and Power Factor : modbus_lib/Complex Power and Power Factor
  Constant1 : Constant  Value=2/60
  Constant2 : Constant  Value=TOC
  Constant3 : Constant  Value=0
  Constant4 : Constant  Value=Ts
  Data Type Conversion{1..7} (7 alike) : DataTypeConversion
  Demux : Demux
  Demux2 : Demux  Outputs=2
  Demux4 : Demux  Outputs=3
  Demux5 : Demux  Outputs=3
  Detect Change : simulink/Logic and Bit Operations/Detect Change  vinit=0  InputProcessing=Inherited  OutDataTypeStr=uint8
  Divide : Product  Inputs=*/
  Gain : Gain  Gain=2^3
  Gain1 : Gain  Gain=100
  Gain10 : Gain  Gain=1/1000
  Gain{3..5,8..9,11..12} (7 alike) : Gain  Gain=10
  Gain13 : Gain  Gain=2
  Gain14 : Gain  Gain=2^14
  Gain{15..20} (6 alike) : Gain  Gain=1.4142
  Gain2 : Gain  Gain=1/VRMSLL
  Gain21 : Gain  Gain=1/(VRMSLL/1.732)
  Gain6 : Gain  Gain=1/1000
  Gain7 : Gain  Gain=1/1000
  Logical Operator : Logic  Operator=NOT  AllPortsSameDT=off  OutDataTypeStr=boolean
  Logical Operator1 : Logic  Operator=OR  AllPortsSameDT=off  OutDataTypeStr=boolean
  Logical Operator4 : Logic  Operator=OR  Inputs=4  AllPortsSameDT=off  OutDataTypeStr=boolean
  Memory{1..3,8..9} (5 alike) : Memory
  Mux : Mux
  Mux1 : Mux  Inputs=7
  Mux2 : Mux  Inputs=2
  PQ_Calculator : Subsystem
  Phase_Calc : Subsystem
  Phase_Calc1 : Subsystem
  R50512759 : modbus_lib/R50512759  VRMSLL=VRMSLL  IOC=IOC  TOC=TOC  Ts=Ts
  RMS_Calculator : Subsystem
  RMS_Calculator1 : Subsystem
  Relay 25 - Sync Check - RS : modbus_lib/Relay 25 - Sync Check - RS  VRMSLL=VRMSLL  Ts=Ts  dV_threshold=dV_threshold  angle_threshold=angle_threshold  dF_threshold=dF_threshold
  Sum : Sum  Inputs=|++
  Sum1 : Sum  Inputs=+++
  Terminator : Terminator
  Terminator1 : Terminator
  Terminator2 : Terminator
  bitwise_faults : Subsystem
  bkr_control : modbus_lib/bkr_control  enable=bkrCtrl_enable  status=bkrCtrl_status
  pf bitwise : Subsystem
  trip_out mng : MATLAB Function  TreatAsAtomicUnit=on
  OUTPUT : Outport
  TO_MODBUS : Outport  Port=2
  wires:
  Demux2/2 -> [op_mode], Logical Operator1/2  "mode"
  [Iabc] -> R50512759/1
  Demux5/3 -> [Vc_rms]
  Demux5/2 -> [Vb_rms]
  Demux5/1 -> [Va_rms]
  Demux4/1 -> [Ia_rms]
  Demux4/2 -> [Ib_rms]
  Demux4/3 -> [Ic_rms]
  RMS_Calculator1/1(RMS_Signal) -> Demux5/1, [Vabc_rms]
  RMS_Calculator/1(RMS_Signal) -> Demux4/1, [Iabc_rms]
  [Vabc] -> RMS_Calculator1/1(Signal)
  [Iabc] -> RMS_Calculator/1(Signal)
  PQ_Calculator/2(Q) -> [Q]
  PQ_Calculator/1(P) -> [P]
  [S] -> Gain7/1
  [Q] -> Gain6/1
  [P] -> Gain10/1
  [Iabc] -> PQ_Calculator/2(Iabc)
  [Vabc] -> PQ_Calculator/1(Vabc)
  [Iabc] -> Bus Creator/1  "Iabc"
  [Vabc] -> Bus Creator/2  "Vabc"
  FROM_MODBUS/1 -> Demux2/1
  Bus Creator1/1 -> TO_MODBUS/1  "sm_in"
  [freq] -> Gain4/1
  [pf] -> Gain1/1
  [P] -> Bus Creator/3  "P"
  [Q] -> Bus Creator/4  "Q"
  [Vabc] -> Gain2/1
  Gain2/1 -> CS Modified PLL/1
  Phase_Calc/1(Phase a) -> [Va_phase]
  Phase_Calc/2(Phase b) -> [Vb_phase]
  Phase_Calc/3(Phase c) -> [Vc_phase]
  [Iabc] -> Divide/1
  Phase_Calc1/1(Phase a) -> [Ia_phase]
  Phase_Calc1/2(Phase b) -> [Ib_phase]
  Phase_Calc1/3(Phase c) -> [Ic_phase]
  Divide/1 -> CS Modified PLL1/1
  Constant2/1 -> Divide/2
  [Vc_phase] -> Gain3/1
  [Vb_phase] -> Gain5/1
  [Va_phase] -> Gain8/1
  [Ic_phase] -> Gain9/1
  [Ib_phase] -> Gain11/1
  [Ia_phase] -> Gain12/1
  [Vabc_rms] -> R50512759/3
  Logical Operator4/1 -> Logical Operator/1, Relay 25 - Sync Check - RS/3
  Logical Operator/1 -> Data Type Conversion1/1
  R50512759/1 -> Logical Operator4/1, [R50]  "50"
  Sum1/1 -> Memory2/1
  Gain13/1 -> Sum1/2
  Sum/1 -> Memory9/1
  Gain/1 -> Sum/2
  R50512759/2 -> Logical Operator4/2, [R51]  "51"
  [R50] -> Mux/1
  [R51] -> Mux/2
  Mux/1 -> Data Type Conversion4/1
  Demux/1 -> Sum/1
  Demux/2 -> Gain/1
  Demux/3 -> Sum1/1
  Demux/4 -> Gain13/1
  Data Type Conversion4/1 -> Demux/1
  Memory9/1 -> Bus Creator1/24
  Memory2/1 -> Bus Creator1/25
  [Iabc_rms] -> R50512759/2
  [reset] -> R50512759/4
  [op_mode] -> Memory1/1
  Memory8/1 -> [Status], Bus Creator2/2  "Logic_trip"
  Constant1/1 -> trip_out mng/5(synch_check_time)
  Relay 25 - Sync Check - RS/1 -> trip_out mng/2(bool_R25), [R25]  "R25"
  [op_mode] -> trip_out mng/3(op_mode_in)
  Data Type Conversion1/1 -> trip_out mng/4(trip_in)  "trip_in"
  [op_mode] -> Relay 25 - Sync Check - RS/4
  trip_out mng/1(trip_out) -> bkr_control/1
  CS Modified PLL1/2 -> Phase_Calc1/1(wt)
  CS Modified PLL/1 -> [freq]
  CS Modified PLL/2 -> Phase_Calc/1(wt)
  CS Modified PLL1/1 -> Terminator1/1
  CS Modified PLL1/3 -> Terminator2/1
  CS Modified PLL/3 -> Terminator/1
  [freq] -> Bus Creator/5  "freq"
  [Va_rms] -> Bus Creator/6  "Va_rms"
  [pf] -> Bus Creator/7  "pf"
  [Ia_mag] -> Bus Creator1/1
  Gain12/1 -> Bus Creator1/2
  [Ib_mag] -> Bus Creator1/3
  Gain11/1 -> Bus Creator1/4
  [Ic_mag] -> Bus Creator1/5
  Gain9/1 -> Bus Creator1/6
  [Ia_rms] -> Bus Creator1/7
  [Ib_rms] -> Bus Creator1/8
  [Ic_rms] -> Bus Creator1/9
  [Va_rms] -> Bus Creator1/10
  [Vb_rms] -> Bus Creator1/11
  [Vc_rms] -> Bus Creator1/12
  [Va_mag] -> Bus Creator1/13
  Gain8/1 -> Bus Creator1/14
  [Vb_mag] -> Bus Creator1/15
  Gain5/1 -> Bus Creator1/16
  [Vc_mag] -> Bus Creator1/17
  Gain3/1 -> Bus Creator1/18
  Gain10/1 -> Bus Creator1/19
  Gain6/1 -> Bus Creator1/20
  Gain7/1 -> Bus Creator1/21
  Gain1/1 -> Bus Creator1/22
  Gain4/1 -> Bus Creator1/23
  Data Type Conversion2/1 -> Gain14/1
  [Status] -> Data Type Conversion2/1
  [Vabc] -> Relay 25 - Sync Check - RS/1
  [Ia_rms] -> Gain15/1
  [Ib_rms] -> Gain16/1
  [Ic_rms] -> Gain17/1
  [Va_rms] -> Gain18/1
  [Vb_rms] -> Gain19/1
  [Vc_rms] -> Gain20/1
  Gain20/1 -> [Vc_mag]
  Gain19/1 -> [Vb_mag]
  Gain18/1 -> [Va_mag]
  Gain17/1 -> [Ic_mag]
  Gain16/1 -> [Ib_mag]
  Gain15/1 -> [Ia_mag]
  [Va_rms] -> Gain21/1
  Gain21/1 -> Bus Creator/8  "Vpu"
  Constant4/1 -> trip_out mng/1(Ts)
  bkr_control/1 -> Memory8/1
  R50512759/3 -> [R27]  "27"
  R50512759/4 -> [R59]  "59"
  Mux1/1 -> bitwise_faults/1(S)
  bitwise_faults/1(s) -> Bus Creator/9  "status"
  [reset] -> Data Type Conversion5/1
  [Status] -> Data Type Conversion6/1
  [R25] -> Mux1/2  "R25_Sync"
  [R27] -> Mux1/3  "R27_Under Voltage"
  [R50] -> Mux1/4  "R50_Instant_OverCurrent"
  [R51] -> Mux1/5  "R51_Time_OverCurrent"
  [R59] -> Mux1/6  "R59_Over_Voltage"
  Data Type Conversion5/1 -> Mux1/7  "reset"
  Data Type Conversion6/1 -> Mux1/1  "Status"
  [Vabc_line] -> Relay 25 - Sync Check - RS/2
  Bus Selector1/1 -> [Iabc]  "<Iabc>"
  Bus Selector1/2 -> [Vabc]  "<Vabc_bus>"
  Bus Selector1/3 -> [Vabc_line]  "<Vabc_line>"
  MEASUREMENTS/1 -> Bus Selector1/1
  Bus Creator/1 -> Memory3/1
  Memory1/1 -> Bus Creator2/1  "op_mode"
  Bus Creator2/1 -> OUTPUT/1
  [P] -> Complex Power and Power Factor/1
  [Q] -> Complex Power and Power Factor/2
  Complex Power and Power Factor/1 -> [S]
  Complex Power and Power Factor/2 -> [pf]
  Complex Power and Power Factor/3 -> [exp_imp]
  Complex Power and Power Factor/4 -> [lag_lead]
  [R27] -> Mux/3
  [R59] -> Mux/4
  Gain14/1 -> Sum1/3
  Mux2/1 -> Data Type Conversion3/1
  pf bitwise/1(s) -> Bus Creator/10  "pf_states"
  [exp_imp] -> Mux2/1
  [lag_lead] -> Mux2/2
  Memory3/1 -> Bus Creator2/3  "m"
  Data Type Conversion3/1 -> pf bitwise/1(S)
  Demux2/1 -> Logical Operator1/1  "reset"
  Logical Operator1/1 -> Detect Change/1
  Detect Change/1 -> [reset]  "reset"
  Data Type Conversion7/1 -> Logical Operator4/3, Logical Operator4/4
  Constant3/1 -> Data Type Conversion7/1

== system modbus_lib/bkr_control ==
  note: The default condition of this block is Enable=0
  note: This control is only valid for system relays.
      | It does not control the woodward breakers
  note: Bkr_control
      | 1-Closed
      | 0-Open
  note: The signal trip_out is active when Enable=0.
  Trip_in : Inport
  Digital Clock : DigitalClock  SampleTime=Ts
  MATLAB Function : MATLAB Function  TreatAsAtomicUnit=on
  bkr_control : Constant  Value=status
  enable_control : Constant  Value=enable
  Trip_out : Outport
  wires:
  MATLAB Function/1(logic_out) -> Trip_out/1
  Trip_in/1 -> MATLAB Function/1(trip_in)
  enable_control/1 -> MATLAB Function/2(enable)
  bkr_control/1 -> MATLAB Function/3(status)
  Digital Clock/1 -> MATLAB Function/4(time)

== system modbus_lib/BATT_MODBUS/bitwise_faults ==
  note: Constant array has LSB on most left.
  batt_fault : Inport
  Bitwise Operator : simulink/Logic and Bit Operations/Bitwise Operator  logicop=OR  UseBitMask=off  NumInputPorts=8  BitMask=bin2dec('11011001')  BitMaskRealWorld=Stored Integer
  Data Type Conversion : DataTypeConversion  OutDataTypeStr=uint16
  Data Type Conversion1 : DataTypeConversion
  Demux : Demux  Outputs=8
  Shift Arithmetic : ArithShift  BitShiftNumber=1  BitShiftDirection=Left
  Shift Arithmetic1 : ArithShift  BitShiftNumber=2  BitShiftDirection=Left
  Shift Arithmetic2 : ArithShift  BitShiftNumber=3  BitShiftDirection=Left
  Shift Arithmetic3 : ArithShift  BitShiftNumber=4  BitShiftDirection=Left
  Shift Arithmetic4 : ArithShift  BitShiftNumber=5  BitShiftDirection=Left
  Shift Arithmetic5 : ArithShift  BitShiftNumber=6  BitShiftDirection=Left
  Shift Arithmetic6 : ArithShift  BitShiftNumber=7  BitShiftDirection=Left
  to_mb : Outport
  wires:
  Shift Arithmetic6/1 -> Bitwise Operator/8
  Shift Arithmetic5/1 -> Bitwise Operator/7
  Shift Arithmetic4/1 -> Bitwise Operator/6
  Shift Arithmetic3/1 -> Bitwise Operator/5
  Shift Arithmetic2/1 -> Bitwise Operator/4
  Shift Arithmetic1/1 -> Bitwise Operator/3
  Shift Arithmetic/1 -> Bitwise Operator/2
  Demux/8 -> Shift Arithmetic6/1
  Demux/7 -> Shift Arithmetic5/1
  Data Type Conversion/1 -> Demux/1
  Demux/1 -> Bitwise Operator/1
  Demux/2 -> Shift Arithmetic/1
  Demux/3 -> Shift Arithmetic1/1
  Demux/4 -> Shift Arithmetic2/1
  Demux/5 -> Shift Arithmetic3/1
  Demux/6 -> Shift Arithmetic4/1
  batt_fault/1 -> Data Type Conversion/1
  Bitwise Operator/1 -> Data Type Conversion1/1
  Data Type Conversion1/1 -> to_mb/1

== system modbus_lib/CS Modified PLL/Controller ==
  note: Pierre Giroux, Gilbert Sybille
      | Power System Simulation Laboratory
      | IREQ, Hydro-Quebc
  note: Discrete PID Controller
  Error : Inport
  Discrete Derivative : simulink/Discrete/Discrete Derivative  gainval=1.0  ICPrevScaledInput=0.0  InputProcessing=Inherited  OutMin=[]  OutMax=[]  OutDataType=sfix(16)  OutScaling=2^-10  DoSatur=off
  Discrete-Time Integrator : DiscreteIntegrator  InitialCondition=Init  SampleTime=Ts  LimitOutput=on  UpperSaturationLimit=UpperLimit  LowerSaturationLimit=LowerLimit  ICPrevOutput=DiscIntNeverNeededParam  ICPrevScaledInput=DiscIntNeverNeededParam
  Kp4 : Gain  Gain=Kp  SaturateOnIntegerOverflow=on  OutDataTypeStr=Inherit: Same as input  ParamDataTypeStr=Inherit: Same as input
  Kp5 : Gain  Gain=Ki  SaturateOnIntegerOverflow=on  OutDataTypeStr=Inherit: Same as input  ParamDataTypeStr=Inherit: Same as input
  Kp6 : Gain  Gain=Kd  SaturateOnIntegerOverflow=on  OutDataTypeStr=Inherit: Same as input  ParamDataTypeStr=Inherit: Same as input
  Saturation2 : Saturate  UpperLimit=UpperLimit  LowerLimit=LowerLimit
  Sum6 : Sum  Inputs=+++  SaturateOnIntegerOverflow=on  InputSameDT=on  OutDataTypeStr=Inherit: Same as first input
  Zero-Order Hold : ZeroOrderHold  SampleTime=Ts
  Out : Outport  InitialOutput=0
  wires:
  Error/1 -> Kp4/1, Kp5/1, Kp6/1
  Sum6/1 -> Saturation2/1
  Kp5/1 -> Discrete-Time Integrator/1
  Kp6/1 -> Zero-Order Hold/1
  Kp4/1 -> Sum6/1
  Discrete-Time Integrator/1 -> Sum6/2
  Discrete Derivative/1 -> Sum6/3
  Saturation2/1 -> Out/1
  Zero-Order Hold/1 -> Discrete Derivative/1

== system modbus_lib/Gen_Synch/Freq_Comparator ==
  f_grid : Inport
  f_gen : Inport  Port=2
  Abs : Abs
  Compare To Constant2 : simulink/Logic and Bit Operations/Compare To Constant  relop=<=  const=0.2  OutDataTypeStr=uint8
  Fcn2 : Fcn  Expr=u(2)-u(1)
  Mux1 : Mux  Inputs=2
  Diff : Outport
  Locked : Outport  Port=2
  wires:
  Compare To Constant2/1 -> Locked/1
  f_grid/1 -> Mux1/1
  f_gen/1 -> Mux1/2
  Fcn2/1 -> Diff/1, Abs/1
  Mux1/1 -> Fcn2/1
  Abs/1 -> Compare To Constant2/1
